simulink model "DC_Motor_ControlStrategies"  (R2025a)
settings: Solver=VariableStepAuto  StartTime=0.0  StopTime=3  RelTol=1e-3
undefined symbols (not defined in the file): B_m, J_m, kfi, L_a, R_a, T_e, T_m, T_nl, V_an
libraries: slpidlib x4, spsControlledVoltageSourceLib x2, spsDCMachineLib x2, spspowerguiLib x1
settings Model: Creator=DE MK - EN  LastModifiedBy=Chrisson

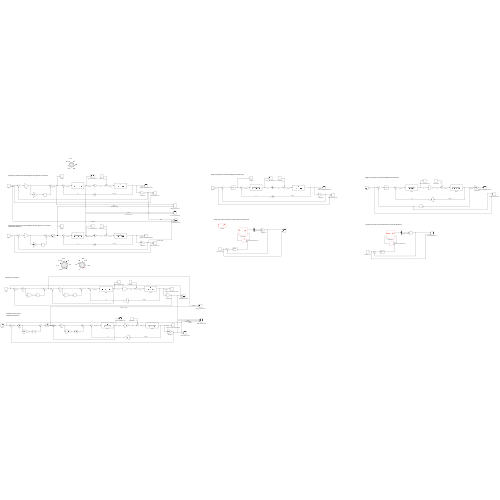
[thumbnail: Simulink's stored preview of the top-level diagram]
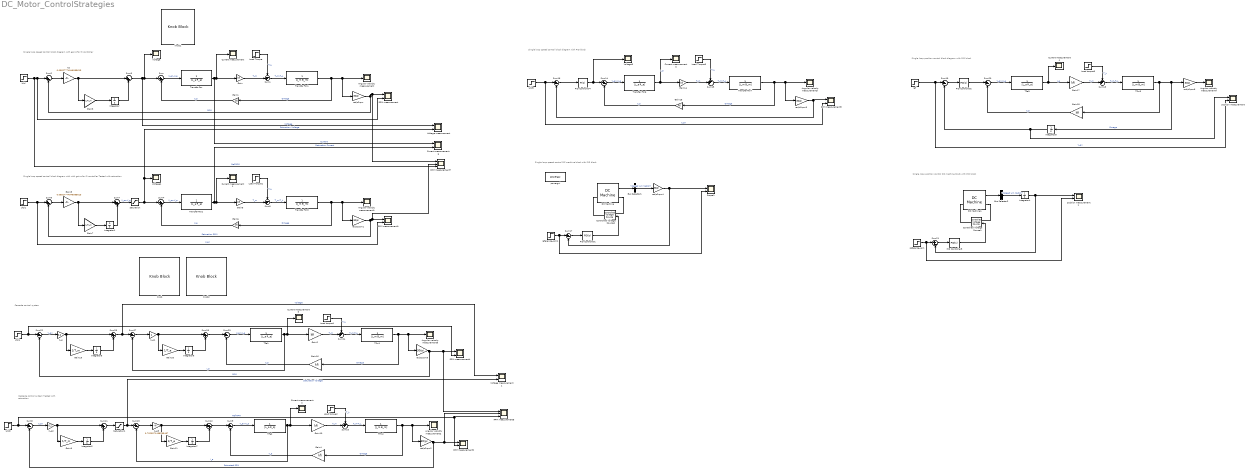
== system DC_Motor_ControlStrategies ==
  note: Single loop speed control block diagram with gains for PI controller
  note: Single loop speed control block diagram with with gains for PI controller
      | Tested with saturation
  note: Single loop speed control block diagram with PID block
  note: Single loop speed control DC machine block with PID block
  note: Single loop position control block diagram with PID block
  note: Single loop position control DC machine block with PID block
  note: Cascade control system
  note: Cascade control system
      | Tested with saturation
  Angular velocity measurement{,1..5} (6 alike) : Scope
      Angular velocity measurement settings: ActiveDisplayYMinimum=-131.91004  ActiveDisplayYMaximum=1187.19039
      Angular velocity measurement1 settings: ActiveDisplayYMinimum=-131.91004  ActiveDisplayYMaximum=1187.19039  DataLoggingVariableName=ScopeData2
      Angular velocity measurement2 settings: ActiveDisplayYMinimum=-105.6703  ActiveDisplayYMaximum=951.03269  DataLoggingVariableName=ScopeData6
      Angular velocity measurement3 settings: ActiveDisplayYMinimum=-131.91004  ActiveDisplayYMaximum=1187.19039  DataLoggingVariableName=ScopeData10
      Angular velocity measurement4 settings: ActiveDisplayYMinimum=-105.6696  ActiveDisplayYMaximum=951.02642  DataLoggingVariableName=ScopeData14
      Angular velocity measurement5 settings: ActiveDisplayYMinimum=-105.6703  ActiveDisplayYMaximum=951.03269  DataLoggingVariableName=ScopeData18
  Bus Selector1 : BusSelector  OutputSignals=Speed wm (rad/s)
  Bus Selector2 : BusSelector  OutputSignals=Speed wm (rad/s)
  Controlled Voltage Source1 : spsControlledVoltageSourceLib/Controlled Voltage Source  Initialize=on  Source_Type=DC  Amplitude=0  Phase=0  Frequency=0  Measurements=None
  Controlled Voltage Source2 : spsControlledVoltageSourceLib/Controlled Voltage Source  Initialize=on  Source_Type=DC  Amplitude=V_an  Phase=0  Frequency=0  Measurements=None
  Current measurement{,1..5} (6 alike) : Scope
      Current measurement settings: Title=Motor Current  ActiveDisplayYMinimum=-0.0869  ActiveDisplayYMaximum=0.43656  YLabel=Current(A)
      Current measurement1 settings: Title=Motor Current  ActiveDisplayYMinimum=-1.34352  ActiveDisplayYMaximum=6.66329  YLabel=Current(A)  DataLoggingVariableName=ScopeData3
      Current measurement2 settings: ActiveDisplayYMinimum=-0.50986  ActiveDisplayYMaximum=4.58876  DataLoggingVariableName=ScopeData7
      Current measurement3 settings: Title=Motor Current  ActiveDisplayYMinimum=-0.00098  ActiveDisplayYMaximum=0.00882  YLabel=Current(A)  DataLoggingVariableName=ScopeData11
      Current measurement4 settings: ActiveDisplayYMinimum=-392.57944  ActiveDisplayYMaximum=1728.55987  DataLoggingVariableName=ScopeData15
      Current measurement5 settings: ActiveDisplayYMinimum=-0.50986  ActiveDisplayYMaximum=4.58876  DataLoggingVariableName=ScopeData19
  Current measurement6 : Scope  NumInputPorts=2
      settings: Title=Current of DC motor  ActiveDisplayYMinimum=-1.81191  ActiveDisplayYMaximum=9.10178  YLabel=Current(A)  DataLoggingVariableName=ScopeData22
  DC Machine : spsDCMachineLib/DC Machine  PresetModel=No  MechanicalLoad=Torque TL  FieldType=Permanent magnet  ShowDetailedParameters=on  MeasurementBus=off  RLa=[R_a L_a]  RLf=[180 71.47]  Laf=0.6458  MachineConstant=Torque constant (N.m/A)  Ke=1.8  Kt=kfi  J=J_m  Bm=B_m  Tf=0  w0=0  Ifinit=1  TsPowergui=0  TsBlock=-1
  DC Machine1 : spsDCMachineLib/DC Machine  PresetModel=No  MechanicalLoad=Torque TL  FieldType=Permanent magnet  ShowDetailedParameters=on  MeasurementBus=off  RLa=[R_a L_a]  RLf=[180 71.47]  Laf=0.6458  MachineConstant=Torque constant (N.m/A)  Ke=1.8  Kt=kfi  J=J_m  Bm=B_m  Tf=0  w0=0  Ifinit=1  TsPowergui=0  TsBlock=-1
  Gain{,1..2,4..6,10,14..18} (12 alike) : Gain  Gain=kfi
  Gain11 : Gain  Gain=1/T_e
  Gain{3,7,9,19} (4 alike) : Gain  Gain=1/T_m
  Gain20 : Gain  Gain=1/T_e
  Gain8 : Gain  Gain=0.09527774946085613
  Integrator{,1..7} (8 alike) : Integrator
  K_p : Gain  Gain=0.2
  K_p1 : Gain
  K_p2 : Gain  Gain=0.2
  K_p3 : Gain  Gain=0.7020371438293457
  Knob : KnobBlock  ScaleMin=0.0001  ScaleMax=0.2
  Knob1 : KnobBlock  ScaleMin=0.0001  ScaleMax=0.2
  Knob2 : KnobBlock  ScaleMin=0.0001  ScaleMax=1
  Kp : Gain  Gain=0.09527774946085613
  Load Torque : Step  Time=2  After=T_nl  SampleTime=0
  Load Torque1 : Step  Time=2  After=T_nl  SampleTime=0
  Load Torque3 : Step  Time=2  After=T_nl  SampleTime=0
  Load torque1 : Step  Time=2  After=T_nl  SampleTime=0
  Load torque2 : Step  Time=2  After=T_nl  SampleTime=0
  Load torque3 : Step  Time=2  After=T_nl  SampleTime=0
  PID Controller1 : slpidlib/PID Controller  Controller=PID  Form=Parallel  TimeDomain=Continuous-time  UseExternalTs=off  SampleTime=-1  IntegratorMethod=Forward Euler  FilterMethod=Forward Euler  ControllerParametersSource=internal  P=0.018216850136936  I=3.35111284474081  UseKiTs=off  D=-2.65817085568045e-06  UseExternalDerivativeSource=off  N=6853.15245933383  UseFilter=on  TunerSelectOption=Transfer Function Based (PID Tuner App)  InitialConditionSource=internal  InitialConditionForIntegrator=0  InitialConditionForFilter=0  DifferentiatorICPrevScaledInput=0  ExternalReset=none  TrackingMode=off  Kt=1  LimitOutput=off  SatLimitsSource=internal  UpperSaturationLimit=inf  LowerSaturationLimit=-inf  LinearizeAsGain=on  AntiWindupMode=none  Kb=1  LimitIntegrator=off  UpperIntegratorSaturationLimit=inf  LowerIntegratorSaturationLimit=-inf  POutMin=[]  POutMax=[]  IOutMin=[]  IOutMax=[]  DOutMin=[]  DOutMax=[]  NOutMin=[]  NOutMax=[]  SumOutMin=[]  SumOutMax=[]  SaturationOutMin=[]  SaturationOutMax=[]  PParamMin=[]  PParamMax=[]  IParamMin=[]  IParamMax=[]  DParamMin=[]  DParamMax=[]  NParamMin=[]  NParamMax=[]  KbParamMin=[]  KbParamMax=[]  KtParamMin=[]  KtParamMax=[]  KbOutMin=[]  KbOutMax=[]  KtOutMin=[]  KtOutMax=[]  IntegratorOutMin=[]  IntegratorOutMax=[]  FilterOutMin=[]  FilterOutMax=[]  SumI1OutMin=[]  SumI1OutMax=[]  SumI2OutMin=[]  SumI2OutMax=[]  SumI3OutMin=[]  SumI3OutMax=[]  SumI4OutMin=[]  SumI4OutMax=[]  SumDOutMin=[]  SumDOutMax=[]  DifferentiatorOutMin=[]  DifferentiatorOutMax=[]  FilterDiffOutCoefMin=[]  FilterDiffOutCoefMax=[]  ReciprocalOutMin=[]  ReciprocalOutMax=[]  SumDenOutMin=[]  SumDenOutMax=[]  SumNumOutMin=[]  SumNumOutMax=[]  DivideOutMin=[]  DivideOutMax=[]  UdiffTsProdOutMin=[]  UdiffTsProdOutMax=[]  NTsProdOutMin=[]  NTsProdOutMax=[]  UintegralTsProdOutMin=[]  UintegralTsProdOutMax=[]  UngainTsProdOutMin=[]  UngainTsProdOutMax=[]  ClampingZeroOutDataTypeStr=Inherit: Inherit via back propagation  ClampingZeroOutMin=[]  ClampingZeroOutMax=[]  FilterDenConstantOutDataTypeStr=Inherit: Inherit via back propagation  FilterDenConstantOutMin=[]  FilterDenConstantOutMax=[]  PCopyOutDataTypeStr=Inherit: Inherit via back propagation  PCopyOutMin=[]  PCopyOutMax=[]  NCopyOutDataTypeStr=Inherit: Inherit via back propagation  NCopyOutMin=[]  NCopyOutMax=[]  IntegratorContinuousStateAttributes=''  IntegratorStateMustResolveToSignalObject=off  IntegratorRTWStateStorageClass=Auto  FilterContinuousStateAttributes=''  FilterStateMustResolveToSignalObject=off  FilterRTWStateStorageClass=Auto  ParallelPVariant=InternalParameters  IdealPVariant=Disabled  IVariant=InternalParameters  DVariant=InternalParameters  IntegratorVariant=Continuous  SatVariant=Disabled  AWVariant=Passthrough  PCopyVariant=Disabled  TRVariant=Disabled  FdbkBlocksVariant=Forward  IdealPFdbkVariant=Disabled  SatFdbkVariant=Disabled  DerivativeFilterVariant=ContFilter  NVariant=InternalParameters  NCopyVariant=Disabled  FilterICVariant=InternalICsFilter  IntegratorICVariant=InternalICs  ExternalResetVariant=Disabled  TRSumVariant=Passthrough  SumFdbkVariant=Disabled  SumVariant=Sum_PID  TsampFilterVariant=InternalTs  TsampNgainVariant=Passthrough  TsampIntegralVariant=Disabled_SignalSpec  ExternalSaturationOutDataTypeStr=Inherit: Same as second input  DerivativeSourceVariant=ErrorSignal  PreIntVariant=InternalPreInt
  PID Controller2 : slpidlib/PID Controller  Controller=PID  Form=Parallel  TimeDomain=Continuous-time  UseExternalTs=off  SampleTime=-1  IntegratorMethod=Forward Euler  FilterMethod=Forward Euler  ControllerParametersSource=internal  P=0.356411764508581  I=1.20490397968824  UseKiTs=off  D=0.0075787229323932  UseExternalDerivativeSource=off  N=2285.65595208321  UseFilter=on  TunerSelectOption=Transfer Function Based (PID Tuner App)  InitialConditionSource=internal  InitialConditionForIntegrator=0  InitialConditionForFilter=0  DifferentiatorICPrevScaledInput=0  ExternalReset=none  TrackingMode=off  Kt=1  LimitOutput=off  SatLimitsSource=internal  UpperSaturationLimit=inf  LowerSaturationLimit=-inf  LinearizeAsGain=on  AntiWindupMode=none  Kb=1  LimitIntegrator=off  UpperIntegratorSaturationLimit=inf  LowerIntegratorSaturationLimit=-inf  POutMin=[]  POutMax=[]  IOutMin=[]  IOutMax=[]  DOutMin=[]  DOutMax=[]  NOutMin=[]  NOutMax=[]  SumOutMin=[]  SumOutMax=[]  SaturationOutMin=[]  SaturationOutMax=[]  PParamMin=[]  PParamMax=[]  IParamMin=[]  IParamMax=[]  DParamMin=[]  DParamMax=[]  NParamMin=[]  NParamMax=[]  KbParamMin=[]  KbParamMax=[]  KtParamMin=[]  KtParamMax=[]  KbOutMin=[]  KbOutMax=[]  KtOutMin=[]  KtOutMax=[]  IntegratorOutMin=[]  IntegratorOutMax=[]  FilterOutMin=[]  FilterOutMax=[]  SumI1OutMin=[]  SumI1OutMax=[]  SumI2OutMin=[]  SumI2OutMax=[]  SumI3OutMin=[]  SumI3OutMax=[]  SumI4OutMin=[]  SumI4OutMax=[]  SumDOutMin=[]  SumDOutMax=[]  DifferentiatorOutMin=[]  DifferentiatorOutMax=[]  FilterDiffOutCoefMin=[]  FilterDiffOutCoefMax=[]  ReciprocalOutMin=[]  ReciprocalOutMax=[]  SumDenOutMin=[]  SumDenOutMax=[]  SumNumOutMin=[]  SumNumOutMax=[]  DivideOutMin=[]  DivideOutMax=[]  UdiffTsProdOutMin=[]  UdiffTsProdOutMax=[]  NTsProdOutMin=[]  NTsProdOutMax=[]  UintegralTsProdOutMin=[]  UintegralTsProdOutMax=[]  UngainTsProdOutMin=[]  UngainTsProdOutMax=[]  ClampingZeroOutDataTypeStr=Inherit: Inherit via back propagation  ClampingZeroOutMin=[]  ClampingZeroOutMax=[]  FilterDenConstantOutDataTypeStr=Inherit: Inherit via back propagation  FilterDenConstantOutMin=[]  FilterDenConstantOutMax=[]  PCopyOutDataTypeStr=Inherit: Inherit via back propagation  PCopyOutMin=[]  PCopyOutMax=[]  NCopyOutDataTypeStr=Inherit: Inherit via back propagation  NCopyOutMin=[]  NCopyOutMax=[]  IntegratorContinuousStateAttributes=''  IntegratorStateMustResolveToSignalObject=off  IntegratorRTWStateStorageClass=Auto  FilterContinuousStateAttributes=''  FilterStateMustResolveToSignalObject=off  FilterRTWStateStorageClass=Auto  ParallelPVariant=InternalParameters  IdealPVariant=Disabled  IVariant=InternalParameters  DVariant=InternalParameters  IntegratorVariant=Continuous  SatVariant=Disabled  AWVariant=Passthrough  PCopyVariant=Disabled  TRVariant=Disabled  FdbkBlocksVariant=Forward  IdealPFdbkVariant=Disabled  SatFdbkVariant=Disabled  DerivativeFilterVariant=ContFilter  NVariant=InternalParameters  NCopyVariant=Disabled  FilterICVariant=InternalICsFilter  IntegratorICVariant=InternalICs  ExternalResetVariant=Disabled  TRSumVariant=Passthrough  SumFdbkVariant=Disabled  SumVariant=Sum_PID  TsampFilterVariant=InternalTs  TsampNgainVariant=Passthrough  TsampIntegralVariant=Disabled_SignalSpec  ExternalSaturationOutDataTypeStr=Inherit: Same as second input  DerivativeSourceVariant=ErrorSignal  PreIntVariant=InternalPreInt
  PID Controller3 : slpidlib/PID Controller  Controller=PID  Form=Parallel  TimeDomain=Continuous-time  UseExternalTs=off  SampleTime=-1  IntegratorMethod=Forward Euler  FilterMethod=Forward Euler  ControllerParametersSource=internal  P=0.356411764508581  I=1.20490397968824  UseKiTs=off  D=0.0075787229323932  UseExternalDerivativeSource=off  N=2285.65595208321  UseFilter=on  TunerSelectOption=Transfer Function Based (PID Tuner App)  InitialConditionSource=internal  InitialConditionForIntegrator=0  InitialConditionForFilter=0  DifferentiatorICPrevScaledInput=0  ExternalReset=none  TrackingMode=off  Kt=1  LimitOutput=off  SatLimitsSource=internal  UpperSaturationLimit=inf  LowerSaturationLimit=-inf  LinearizeAsGain=on  AntiWindupMode=none  Kb=1  LimitIntegrator=off  UpperIntegratorSaturationLimit=inf  LowerIntegratorSaturationLimit=-inf  POutMin=[]  POutMax=[]  IOutMin=[]  IOutMax=[]  DOutMin=[]  DOutMax=[]  NOutMin=[]  NOutMax=[]  SumOutMin=[]  SumOutMax=[]  SaturationOutMin=[]  SaturationOutMax=[]  PParamMin=[]  PParamMax=[]  IParamMin=[]  IParamMax=[]  DParamMin=[]  DParamMax=[]  NParamMin=[]  NParamMax=[]  KbParamMin=[]  KbParamMax=[]  KtParamMin=[]  KtParamMax=[]  KbOutMin=[]  KbOutMax=[]  KtOutMin=[]  KtOutMax=[]  IntegratorOutMin=[]  IntegratorOutMax=[]  FilterOutMin=[]  FilterOutMax=[]  SumI1OutMin=[]  SumI1OutMax=[]  SumI2OutMin=[]  SumI2OutMax=[]  SumI3OutMin=[]  SumI3OutMax=[]  SumI4OutMin=[]  SumI4OutMax=[]  SumDOutMin=[]  SumDOutMax=[]  DifferentiatorOutMin=[]  DifferentiatorOutMax=[]  FilterDiffOutCoefMin=[]  FilterDiffOutCoefMax=[]  ReciprocalOutMin=[]  ReciprocalOutMax=[]  SumDenOutMin=[]  SumDenOutMax=[]  SumNumOutMin=[]  SumNumOutMax=[]  DivideOutMin=[]  DivideOutMax=[]  UdiffTsProdOutMin=[]  UdiffTsProdOutMax=[]  NTsProdOutMin=[]  NTsProdOutMax=[]  UintegralTsProdOutMin=[]  UintegralTsProdOutMax=[]  UngainTsProdOutMin=[]  UngainTsProdOutMax=[]  ClampingZeroOutDataTypeStr=Inherit: Inherit via back propagation  ClampingZeroOutMin=[]  ClampingZeroOutMax=[]  FilterDenConstantOutDataTypeStr=Inherit: Inherit via back propagation  FilterDenConstantOutMin=[]  FilterDenConstantOutMax=[]  PCopyOutDataTypeStr=Inherit: Inherit via back propagation  PCopyOutMin=[]  PCopyOutMax=[]  NCopyOutDataTypeStr=Inherit: Inherit via back propagation  NCopyOutMin=[]  NCopyOutMax=[]  IntegratorContinuousStateAttributes=''  IntegratorStateMustResolveToSignalObject=off  IntegratorRTWStateStorageClass=Auto  FilterContinuousStateAttributes=''  FilterStateMustResolveToSignalObject=off  FilterRTWStateStorageClass=Auto  ParallelPVariant=InternalParameters  IdealPVariant=Disabled  IVariant=InternalParameters  DVariant=InternalParameters  IntegratorVariant=Continuous  SatVariant=Disabled  AWVariant=Passthrough  PCopyVariant=Disabled  TRVariant=Disabled  FdbkBlocksVariant=Forward  IdealPFdbkVariant=Disabled  SatFdbkVariant=Disabled  DerivativeFilterVariant=ContFilter  NVariant=InternalParameters  NCopyVariant=Disabled  FilterICVariant=InternalICsFilter  IntegratorICVariant=InternalICs  ExternalResetVariant=Disabled  TRSumVariant=Passthrough  SumFdbkVariant=Disabled  SumVariant=Sum_PID  TsampFilterVariant=InternalTs  TsampNgainVariant=Passthrough  TsampIntegralVariant=Disabled_SignalSpec  ExternalSaturationOutDataTypeStr=Inherit: Same as second input  DerivativeSourceVariant=ErrorSignal  PreIntVariant=InternalPreInt
  PID Controller4 : slpidlib/PID Controller  Controller=PI  Form=Parallel  TimeDomain=Continuous-time  UseExternalTs=off  SampleTime=-1  IntegratorMethod=Forward Euler  FilterMethod=Forward Euler  ControllerParametersSource=internal  P=0  I=0.0187718415444156  UseKiTs=off  D=0  UseExternalDerivativeSource=off  N=100  UseFilter=on  TunerSelectOption=Transfer Function Based (PID Tuner App)  InitialConditionSource=internal  InitialConditionForIntegrator=0  InitialConditionForFilter=0  DifferentiatorICPrevScaledInput=0  ExternalReset=none  TrackingMode=off  Kt=1  LimitOutput=off  SatLimitsSource=internal  UpperSaturationLimit=inf  LowerSaturationLimit=-inf  LinearizeAsGain=on  AntiWindupMode=none  Kb=1  LimitIntegrator=off  UpperIntegratorSaturationLimit=inf  LowerIntegratorSaturationLimit=-inf  POutMin=[]  POutMax=[]  IOutMin=[]  IOutMax=[]  DOutMin=[]  DOutMax=[]  NOutMin=[]  NOutMax=[]  SumOutMin=[]  SumOutMax=[]  SaturationOutMin=[]  SaturationOutMax=[]  PParamMin=[]  PParamMax=[]  IParamMin=[]  IParamMax=[]  DParamMin=[]  DParamMax=[]  NParamMin=[]  NParamMax=[]  KbParamMin=[]  KbParamMax=[]  KtParamMin=[]  KtParamMax=[]  KbOutMin=[]  KbOutMax=[]  KtOutMin=[]  KtOutMax=[]  IntegratorOutMin=[]  IntegratorOutMax=[]  FilterOutMin=[]  FilterOutMax=[]  SumI1OutMin=[]  SumI1OutMax=[]  SumI2OutMin=[]  SumI2OutMax=[]  SumI3OutMin=[]  SumI3OutMax=[]  SumI4OutMin=[]  SumI4OutMax=[]  SumDOutMin=[]  SumDOutMax=[]  DifferentiatorOutMin=[]  DifferentiatorOutMax=[]  FilterDiffOutCoefMin=[]  FilterDiffOutCoefMax=[]  ReciprocalOutMin=[]  ReciprocalOutMax=[]  SumDenOutMin=[]  SumDenOutMax=[]  SumNumOutMin=[]  SumNumOutMax=[]  DivideOutMin=[]  DivideOutMax=[]  UdiffTsProdOutMin=[]  UdiffTsProdOutMax=[]  NTsProdOutMin=[]  NTsProdOutMax=[]  UintegralTsProdOutMin=[]  UintegralTsProdOutMax=[]  UngainTsProdOutMin=[]  UngainTsProdOutMax=[]  ClampingZeroOutDataTypeStr=Inherit: Inherit via back propagation  ClampingZeroOutMin=[]  ClampingZeroOutMax=[]  FilterDenConstantOutDataTypeStr=Inherit: Inherit via back propagation  FilterDenConstantOutMin=[]  FilterDenConstantOutMax=[]  PCopyOutDataTypeStr=Inherit: Inherit via back propagation  PCopyOutMin=[]  PCopyOutMax=[]  NCopyOutDataTypeStr=Inherit: Inherit via back propagation  NCopyOutMin=[]  NCopyOutMax=[]  IntegratorContinuousStateAttributes=''  IntegratorStateMustResolveToSignalObject=off  IntegratorRTWStateStorageClass=Auto  FilterContinuousStateAttributes=''  FilterStateMustResolveToSignalObject=off  FilterRTWStateStorageClass=Auto  ParallelPVariant=InternalParameters  IdealPVariant=Disabled  IVariant=InternalParameters  DVariant=Disabled  IntegratorVariant=Continuous  SatVariant=Disabled  AWVariant=Passthrough  PCopyVariant=Disabled  TRVariant=Disabled  FdbkBlocksVariant=Forward  IdealPFdbkVariant=Disabled  SatFdbkVariant=Disabled  DerivativeFilterVariant=Disabled  NVariant=Disabled  NCopyVariant=Disabled_SignalSpec  FilterICVariant=Disabled  IntegratorICVariant=InternalICs  ExternalResetVariant=Disabled  TRSumVariant=Passthrough  SumFdbkVariant=Disabled  SumVariant=Sum_PI  TsampFilterVariant=InternalTs  TsampNgainVariant=Passthrough  TsampIntegralVariant=Disabled_SignalSpec  ExternalSaturationOutDataTypeStr=Inherit: Same as second input  DerivativeSourceVariant=Disabled  PreIntVariant=InternalPreInt
  RPM measurement{,1..4} (5 alike) : Scope  NumInputPorts=2
      RPM measurement settings: Title=RPM of DC motor  ActiveDisplayYMinimum=-6.45411  ActiveDisplayYMaximum=58.08702  YLabel=Speed (rpm)  DataLoggingVariableName=ScopeData2
      RPM measurement1 settings: Title=RPM of DC motor  ActiveDisplayYMinimum=-7.31125  ActiveDisplayYMaximum=65.80124  YLabel=Speed (rpm)  DataLoggingVariableName=ScopeData4
      RPM measurement2 settings: Title=RPM of DC motor  ActiveDisplayYMinimum=-229.05802  ActiveDisplayYMaximum=2061.52216  YLabel=Speed (rpm)  DataLoggingVariableName=ScopeData8
      RPM measurement3 settings: Title=RPM of DC motor  ActiveDisplayYMinimum=-125  ActiveDisplayYMaximum=1125  YLabel=Speed (rpm)  DataLoggingVariableName=ScopeData12
      RPM measurement4 settings: Title=RPM of DC motor  ActiveDisplayYMinimum=-229.05802  ActiveDisplayYMaximum=2061.52216  YLabel=Speed (rpm)  DataLoggingVariableName=ScopeData20
  RPM measurement5 : Scope  NumInputPorts=3
      settings: Title=RPM of DC motor  ActiveDisplayYMinimum=-231.25866  ActiveDisplayYMaximum=2081.32793  YLabel=Speed (rpm)  DataLoggingVariableName=ScopeData17
  RPM measurement7 : Scope  NumInputPorts=3
      settings: Title=RPM of DC motor  ActiveDisplayYMinimum=-135.99133  ActiveDisplayYMaximum=1223.92195  YLabel=Speed (rpm)  DataLoggingVariableName=ScopeData23
  Saturation : Saturate  UpperLimit=V_an  LowerLimit=-V_an
  Saturation1 : Saturate  UpperLimit=V_an  LowerLimit=-V_an
  Scope1 : Scope  NumInputPorts=2
      settings: Title=RPM of DC Motor  ActiveDisplayYMinimum=-155.21485  ActiveDisplayYMaximum=1128.36302  YLabel=Speed(RPM)  DataLoggingVariableName=ScopeData13
  Sum{,2,4,6,8..9,13..14,16..17,19..23,27} (16 alike) : Sum  Inputs=|+-
  Sum{1,5,10,15,18,24} (6 alike) : Sum  Inputs=-+|
  Sum{3,7,11..12,25..26} (6 alike) : Sum  Inputs=|++
  TFe1 : TransferFcn  Denominator=[L_a R_a]
  TFe2 : TransferFcn  Denominator=[L_a R_a]
  TFe3 : TransferFcn  Denominator=[L_a R_a]
  TFm1 : TransferFcn  Denominator=[J_m B_m]
  TFm2 : TransferFcn  Denominator=[J_m B_m]
  TFm3 : TransferFcn  Denominator=[J_m B_m]
  Transfer Fcn : TransferFcn  Denominator=[L_a R_a]
  Transfer Fcn1 : TransferFcn  Denominator=[J_m B_m]
  Transfer Fcn2 : TransferFcn  Denominator=[L_a R_a]
  Transfer Fcn3 : TransferFcn  Denominator=[J_m B_m]
  Transfer Fcn6 : TransferFcn  Denominator=[L_a R_a]
  Transfer Fcn7 : TransferFcn  Denominator=[J_m B_m]
  U(s){,1..4} (5 alike) : Step  After=1000  SampleTime=0
  Voltage : Scope
      settings: Title=Motor Voltage  ActiveDisplayYMinimum=-0.75329  ActiveDisplayYMaximum=5.16922  YLabel=Voltage(V)
  Voltage measurement : Scope  NumInputPorts=2
      settings: Title=RPM of DC motor  ActiveDisplayYMinimum=-15.75107  ActiveDisplayYMaximum=107.69685  YLabel=Speed (rpm)  DataLoggingVariableName=ScopeData21
  Voltage measurement1 : Scope  NumInputPorts=2
      settings: Title=Voltage of DC motor  ActiveDisplayYMinimum=-215.12915  ActiveDisplayYMaximum=246.20722  YLabel=Voltage(V)  DataLoggingVariableName=ScopeData26
  Voltage1 : Scope
      settings: Title=Motor Current  ActiveDisplayYMinimum=-7.42049  ActiveDisplayYMaximum=54.15783  YLabel=Current(A)  DataLoggingVariableName=ScopeData5
  Voltage3 : Scope
      settings: Title=Motor Voltage  ActiveDisplayYMinimum=-0.59522  ActiveDisplayYMaximum=5.35698  YLabel=Voltage(V)  DataLoggingVariableName=ScopeData24
  position measurement : Scope  NumInputPorts=2
      settings: Title=Position of DC motor  ActiveDisplayYMinimum=-147.72075  ActiveDisplayYMaximum=1329.48676  YLabel=Position(rad)  DataLoggingVariableName=ScopeData16
  position measurement1 : Scope  NumInputPorts=2
      settings: Title=Position of DC motor  ActiveDisplayYMinimum=-147.72075  ActiveDisplayYMaximum=1329.48676  YLabel=Position(RPM)  DataLoggingVariableName=ScopeData25
  powergui : spspowerguiLib/powergui  Priority=1  SimulationMode=Continuous  SampleTime=50e-6  frequency=60  Iterations=50  frequencyindice=0  Pbase=100e6  ErrMax=1e-4  UnitsV=kV  UnitsW=MW  buscounter=0  FunctionMessages=off  echomessages=off  EnableUseOfTLC=off  CurrentSourceSwitches=off  DisableSnubberDevices=off  DisableRonSwitches=off  DisableVfSwitches=off  DisplayEquations=off  AutomaticDiscreteSolvers=off  SolverType=Tustin/Backward Euler (TBE)  Interpol=off  ExternalGateDelay=off  methode=off  Ts=100  x0status=blocks  SPID=on  SwTol=0  HookPort=off  NonlinearTolerance=1e-4  nMaxIteration=100  ContinueOnMaxIteration=off  RestoreLinks=warning  ResistiveCurrentMeasurement=off  Frange=[0:2:500]  Ylog=off  Xlog=on  ShowGrid=off  save=off  variable=ZData  structure=0  ZoomFFT=off  StartTime=0.0  cycles=1  DisplayStyle=1  fundamental=60  FreqAxis=off  MaxFrequency=1000  frequencyindicesteady=1  RmsSteady=1  display=off
  rad/s2rpm{,1..6} (7 alike) : Gain  Gain=30/pi
  ref : Step  After=1000  SampleTime=0
  reference_rpm : Step  After=1000  SampleTime=0
  reference_rpm1 : Step  After=1000  SampleTime=0
  wires:
  Sum/1 -> Transfer Fcn/1  "V_an-V_a"
  Transfer Fcn/1 -> Current measurement6/1, Current measurement/1, Gain/1  "Current"
  Transfer Fcn1/1 -> rad/s2rpm/1, Angular velocity measurement/1, Gain1/1  "Omega"
  Gain1/1 -> Sum/2  "V_a"
  Load Torque/1 -> Sum1/1  "T_L"
  Sum1/1 -> Transfer Fcn1/1  "T_m-T_L"
  Gain/1 -> Sum1/2  "T_m"
  rad/s2rpm/1 -> Sum2/2, RPM measurement7/1, RPM measurement/1  "RPM"
  U(s)/1 -> RPM measurement7/3, RPM measurement/2, Sum2/1  "Ref RPM"
  Sum3/1 -> Voltage measurement/1, Voltage/1, Sum/1  "Voltage"
  Gain3/1 -> Integrator/1
  Integrator/1 -> Sum3/2
  Kp/1 -> Gain3/1, Sum3/1
  Sum2/1 -> Kp/1
  Gain8/1 -> Sum7/1, Gain7/1
  Sum7/1 -> Saturation/1  "V_an-V_a"
  Sum6/1 -> Gain8/1
  Integrator1/1 -> Sum7/2
  U(s)1/1 -> RPM measurement1/2, Sum6/1  "V_an"
  Load Torque1/1 -> Sum5/1  "T_L"
  Sum5/1 -> Transfer Fcn3/1  "T_m-T_L"
  rad/s2rpm1/1 -> Sum6/2, RPM measurement7/2, RPM measurement1/1  "Saturation RPM"
  Gain5/1 -> Sum5/2  "T_m"
  Sum4/1 -> Transfer Fcn2/1  "V_an-V_a"
  Gain7/1 -> Integrator1/1
  Transfer Fcn3/1 -> rad/s2rpm1/1, Angular velocity measurement1/1, Gain6/1  "Omega"
  Gain6/1 -> Sum4/2  "V_a"
  Transfer Fcn2/1 -> Current measurement6/2, Current measurement1/1, Gain5/1  "Saturation Current"
  Saturation/1 -> Voltage measurement/2, Voltage1/1, Sum4/1  "Saturation Voltage"
  Sum16/1 -> PID Controller4/1
  U(s)3/1 -> RPM measurement3/2, Sum16/1  "V_an"
  Load Torque3/1 -> Sum15/1  "T_L"
  Sum15/1 -> Transfer Fcn7/1  "T_m-T_L"
  rad/s2rpm3/1 -> Sum16/2, RPM measurement3/1
  Gain14/1 -> Sum15/2  "T_m"
  Sum14/1 -> Transfer Fcn6/1  "V_an-V_a"
  Transfer Fcn7/1 -> rad/s2rpm3/1, Angular velocity measurement3/1, Gain15/1  "Omega"
  Gain15/1 -> Sum14/2  "V_a"
  Transfer Fcn6/1 -> Current measurement3/1, Gain14/1  "I_a"
  PID Controller4/1 -> Voltage3/1, Sum14/1
  PID Controller2/1 -> Sum20/1
  Gain18/1 -> Sum20/2  "V_a"
  Sum20/1 -> TFe3/1  "V_an-V_a"
  Sum19/1 -> PID Controller2/1
  Sum18/1 -> TFm3/1  "T_m-T_L"
  Load torque3/1 -> Sum18/1  "T_L"
  TFm3/1 -> rad/s2rpm6/1, Integrator3/1, Gain18/1  "Omega"
  TFe3/1 -> Gain17/1, Current measurement4/1  "I_a"
  Integrator3/1 -> position measurement/1, Sum19/2
  Gain17/1 -> Sum18/2  "T_m"
  ref/1 -> position measurement/2, Sum19/1  "V_an"
  Integrator4/1 -> position measurement1/1, Sum21/2
  Sum21/1 -> PID Controller3/1
  DC Machine1/1 -> Bus Selector2/1
  PID Controller3/1 -> Controlled Voltage Source1/1
  reference_rpm/1 -> position measurement1/2, Sum21/1
  Bus Selector2/1 -> Integrator4/1  "<Speed wm (rad/s)>"
  rad/s2rpm4/1 -> Scope1/1, Sum17/2
  DC Machine/1 -> Bus Selector1/1
  reference_rpm1/1 -> Scope1/2, Sum17/1
  PID Controller1/1 -> Controlled Voltage Source2/1
  Bus Selector1/1 -> rad/s2rpm4/1  "<Speed wm (rad/s)>"
  Sum17/1 -> PID Controller1/1
  K_p/1 -> Gain19/1, Sum25/1
  TFe1/1 -> Sum27/2, Gain2/1, Current measurement5/1  "I_a"
  Sum24/1 -> TFm1/1  "T_m-T_L"
  Sum23/1 -> TFe1/1  "V_an-V_a"
  U(s)4/1 -> RPM measurement4/2, Sum22/1
  Integrator5/1 -> Sum25/2
  Gain19/1 -> Integrator5/1
  Gain2/1 -> Sum24/2  "T_m"
  Sum22/1 -> K_p/1  "V_an"
  TFm1/1 -> rad/s2rpm5/1, Angular velocity measurement5/1, Gain16/1  "Omega"
  Load torque1/1 -> Sum24/1  "T_L"
  Gain16/1 -> Sum23/2  "V_a"
  rad/s2rpm5/1 -> Sum22/2, RPM measurement5/1, RPM measurement4/1  "RPM"
  Integrator6/1 -> Sum26/2
  K_p1/1 -> Sum26/1, Gain20/1
  Gain20/1 -> Integrator6/1
  Sum26/1 -> Sum23/1
  Sum25/1 -> Voltage measurement1/1, Sum27/1  "Voltage"
  Sum27/1 -> K_p1/1
  rad/s2rpm6/1 -> Angular velocity measurement4/1
  K_p3/1 -> Sum12/1, Gain11/1
  Integrator7/1 -> Sum12/2
  Sum12/1 -> Sum9/1
  rad/s2rpm2/1 -> Sum8/2, RPM measurement5/2, RPM measurement2/1  "Saturated RPM"
  Gain4/1 -> Sum9/2  "V_a"
  Integrator2/1 -> Sum11/2
  Sum8/1 -> K_p2/1  "V_an"
  Gain10/1 -> Sum10/2  "T_m"
  Load torque2/1 -> Sum10/1  "T_L"
  Gain9/1 -> Integrator2/1
  K_p2/1 -> Gain9/1, Sum11/1
  Sum10/1 -> TFm2/1  "T_m-T_L"
  Sum13/1 -> K_p3/1
  Sum9/1 -> TFe2/1  "V_an-V_a"
  TFe2/1 -> Sum13/2, Gain10/1, Current measurement2/1  "I_a"
  TFm2/1 -> rad/s2rpm2/1, Angular velocity measurement2/1, Gain4/1  "Omega"
  U(s)2/1 -> RPM measurement5/3, RPM measurement2/2, Sum8/1  "Ref RPM"
  Gain11/1 -> Integrator7/1
  Sum11/1 -> Saturation1/1
  Saturation1/1 -> Voltage measurement1/2, Sum13/1  "Saturation Voltage"
  connections:
  Controlled Voltage Source1/RConn1 -- DC Machine1/LConn1
  DC Machine1/RConn1 -- Controlled Voltage Source1/LConn1
  DC Machine/RConn1 -- Controlled Voltage Source2/LConn1
  Controlled Voltage Source2/RConn1 -- DC Machine/LConn1
